simulink subsystem "SpaceRobot_Model"  (R2022a)
settings: Solver=VariableStepAuto  StartTime=0.0  StopTime=10.0  RelTol=1e-3
model mask{spaceRobot=sc, jointCstr=on, q_0=spaceRobot.q, q_dot_0=spaceRobot.q_dot}
  mask prompts: jointCstr "Apply joint constraints?"; q_0 "Config"; q_dot_0 "Speed"
settings Model: Creator=charl  LastModifiedBy=charl

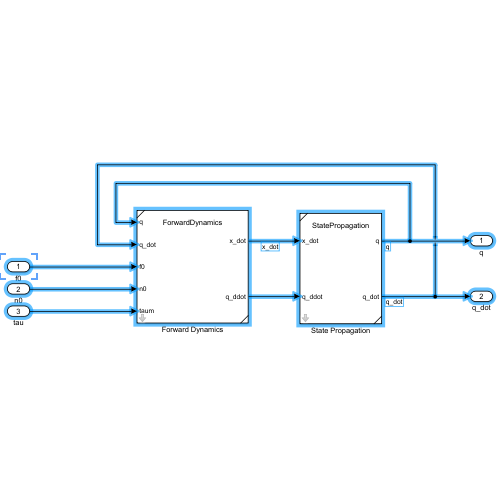
[thumbnail: Simulink's stored preview of the top-level diagram]
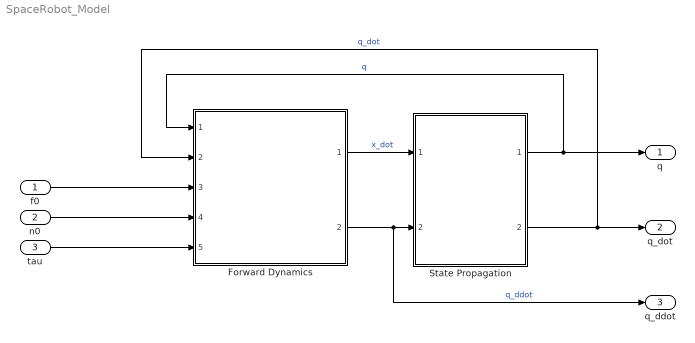
== system SpaceRobot_Model ==
  f0 : Inport
  n0 : Inport  Port=2
  tau : Inport  Port=3
  Forward Dynamics : Subsystem  ReferencedSubsystem=ForwardDynamics  spaceRobot=spaceRobot  SimulateUsing=Interpreted execution
  State Propagation : Subsystem  ReferencedSubsystem=StatePropagation  spaceRobot=spaceRobot  jointCstr=off  q_0=q_0  q_dot_0=q_dot_0
  q : Outport
  q_dot : Outport  Port=2
  q_ddot : Outport  Port=3
  wires:
  f0/1 -> Forward Dynamics/3
  State Propagation/1 -> q/1, Forward Dynamics/1  "q"
  State Propagation/2 -> q_dot/1, Forward Dynamics/2  "q_dot"
  n0/1 -> Forward Dynamics/4
  Forward Dynamics/1 -> State Propagation/1  "x_dot"
  tau/1 -> Forward Dynamics/5
  Forward Dynamics/2 -> State Propagation/2, q_ddot/1  "q_ddot"
